simulink model "Parte2_Controlador"  (R2024a)
settings: Solver=VariableStepAuto  StartTime=0.0  StopTime=20  RelTol=1e-3
settings Model: Creator=salio  LastModifiedBy=Marco
settings SolverCC: MaxConsecutiveMinStep=10  ZeroCrossAlgorithm=Adaptive
settings OptimizationCC: ReuseModelBlockBuffer=off
settings DebuggingCC: SignalInfNanChecking=error  IgnoredZcDiagnostic=none
settings RTWCC: GPUComputeCapability=3.5

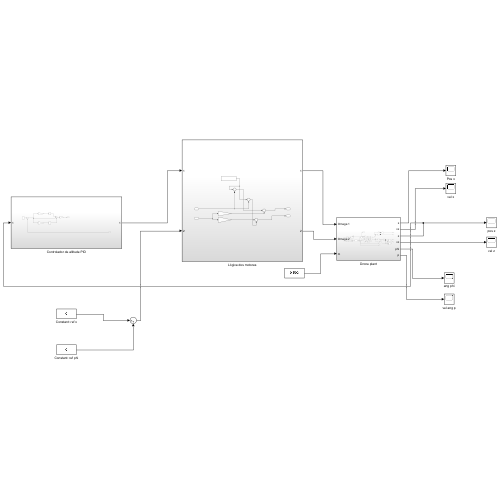
[thumbnail: Simulink's stored preview of the top-level diagram]
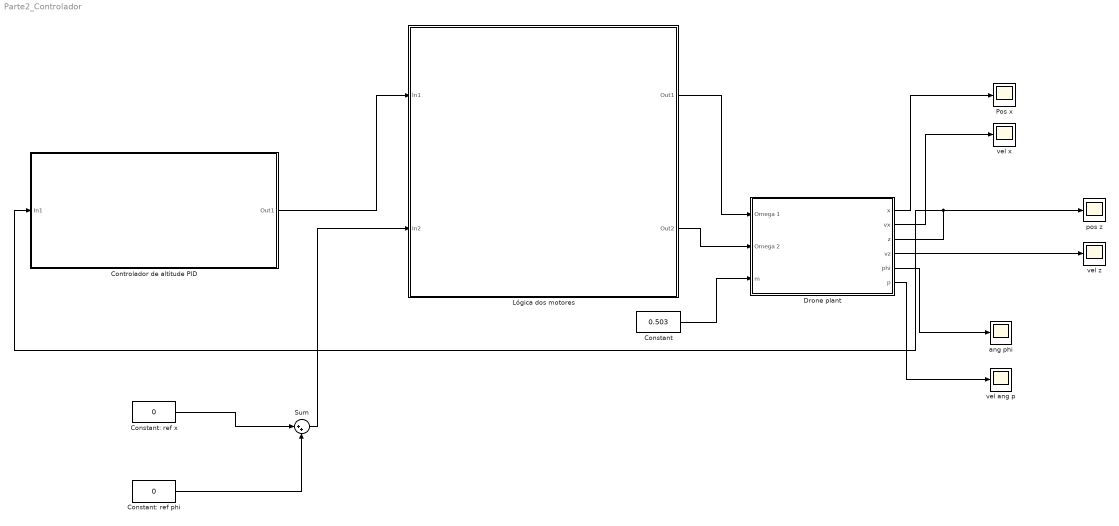
== system Parte2_Controlador ==
  Constant : Constant  Value=0.503
  Constant: ref phi : Constant  Value=0
  Constant: ref x : Constant  Value=0
  Controlador de altitude PID : Subsystem
  Drone plant : Subsystem
  Lógica dos motores : Subsystem
  Pos x : Scope
  Sum : Sum  Inputs=|++
  ang phi : Scope
  pos z : Scope
  vel ang p : Scope
  vel x : Scope
  vel z : Scope
  wires:
  Constant/1 -> Drone plant/3(m)
  Drone plant/1(x) -> Pos x/1
  Drone plant/2(vx) -> vel x/1
  Drone plant/5(phi) -> ang phi/1
  Drone plant/6(p) -> vel ang p/1
  Drone plant/3(z) -> Controlador de altitude PID/1(In1), pos z/1
  Drone plant/4(vz) -> vel z/1
  Sum/1 -> Lógica dos motores/2(In2)
  Lógica dos motores/1(Out1) -> Drone plant/1(Omega 1)
  Lógica dos motores/2(Out2) -> Drone plant/2(Omega 2)
  Controlador de altitude PID/1(Out1) -> Lógica dos motores/1(In1)
  Constant: ref x/1 -> Sum/1
  Constant: ref phi/1 -> Sum/2

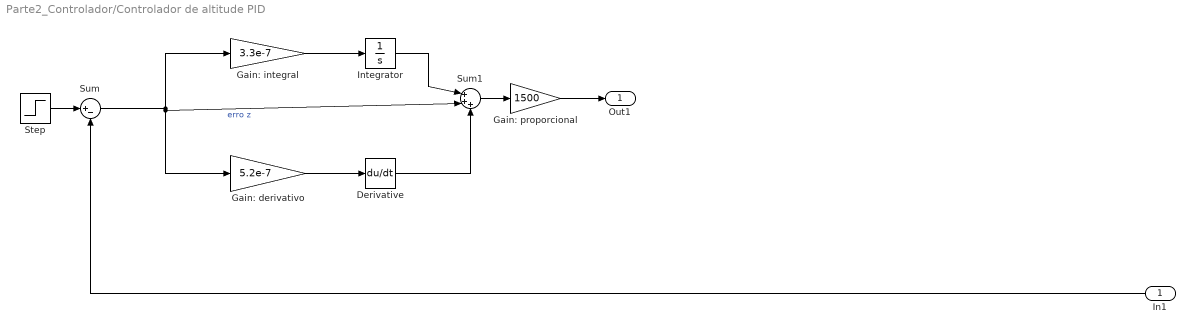
== system Parte2_Controlador/Controlador de altitude PID ==
  In1 : Inport
  Derivative : Derivative
  Gain: derivativo : Gain  Gain=5.2e-7
  Gain: integral : Gain  Gain=3.3e-7
  Gain: proporcional : Gain  Gain=1500
  Integrator : Integrator
  Step : Step  After=5  SampleTime=0
  Sum : Sum  Inputs=|+-
  Sum1 : Sum  Inputs=|+++
  Out1 : Outport
  wires:
  In1/1 -> Sum/2
  Step/1 -> Sum/1
  Gain: integral/1 -> Integrator/1
  Sum/1 -> Gain: derivativo/1, Sum1/2, Gain: integral/1  "erro z"
  Gain: derivativo/1 -> Derivative/1
  Integrator/1 -> Sum1/1
  Derivative/1 -> Sum1/3
  Sum1/1 -> Gain: proporcional/1
  Gain: proporcional/1 -> Out1/1

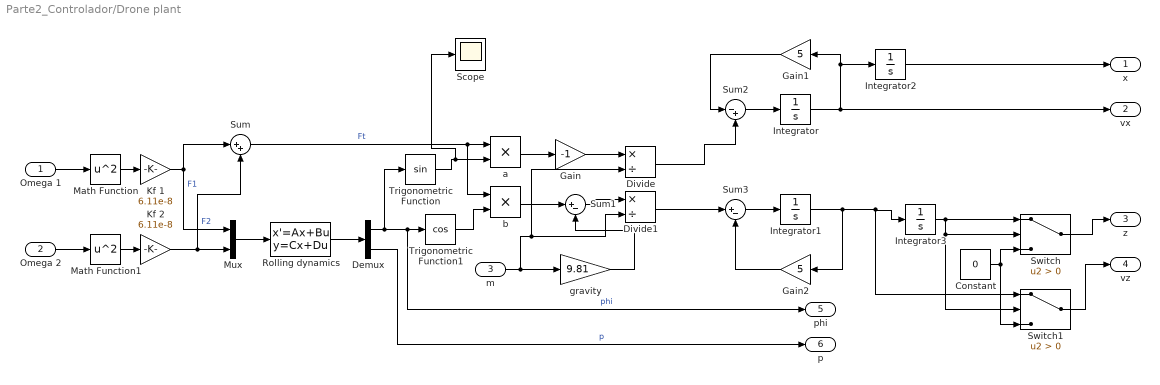
== system Parte2_Controlador/Drone plant ==
  Omega 1 : Inport
  Omega 2 : Inport  Port=2
  m : Inport  Port=3
  Constant : Constant  Value=0
  Demux : Demux  Outputs=2
  Divide : Product  Inputs=*/
  Divide1 : Product  Inputs=*/
  Gain : Gain  Gain=-1
  Gain1 : Gain  Gain=5
  Gain2 : Gain  Gain=5
  Integrator{,1..3} (4 alike) : Integrator
  Kf 1 : Gain  Gain=6.11e-8
  Kf 2 : Gain  Gain=6.11e-8
  Math Function : Math  Operator=square
  Math Function1 : Math  Operator=square
  Mux : Mux  Inputs=2
  Rolling dynamics : StateSpace  A=[0 1; 0 -1800]  B=[0 0; 110.8 -110.8]  C=[1 0; 0 1]  D=[0 0; 0 0]  InitialCondition=0
  Scope : Scope
  Sum : Sum  Inputs=|++
  Sum1 : Sum  Inputs=|+-
  Sum2 : Sum  Inputs=|-+
  Sum3 : Sum  Inputs=|+-
  Switch : Switch  Criteria=u2 > Threshold  SaturateOnIntegerOverflow=off  InputSameDT=off
  Switch1 : Switch  Criteria=u2 > Threshold  SaturateOnIntegerOverflow=off  InputSameDT=off
  Trigonometric Function : Trigonometry
  Trigonometric Function1 : Trigonometry  Operator=cos
  a : Product
  b : Product
  gravity : Gain  Gain=9.81
  x : Outport
  vx : Outport  Port=2
  z : Outport  Port=3
  vz : Outport  Port=4
  phi : Outport  Port=5
  p : Outport  Port=6
  wires:
  Demux/1 -> phi/1, Trigonometric Function1/1, Trigonometric Function/1  "phi"
  Omega 2/1 -> Math Function1/1
  Kf 2/1 -> Mux/2, Sum/2  "F2"
  Kf 1/1 -> Mux/1, Sum/1  "F1"
  Demux/2 -> p/1  "p"
  Trigonometric Function/1 -> Scope/1, a/2
  Math Function/1 -> Kf 1/1
  Omega 1/1 -> Math Function/1
  Mux/1 -> Rolling dynamics/1
  Rolling dynamics/1 -> Demux/1
  Sum/1 -> b/1, a/1  "Ft"
  Trigonometric Function1/1 -> b/2
  Math Function1/1 -> Kf 2/1
  Switch/1 -> z/1
  a/1 -> Gain/1
  Gain/1 -> Divide/1
  Divide/1 -> Sum2/2
  Integrator2/1 -> x/1
  Divide1/1 -> Sum3/1
  Integrator3/1 -> Switch1/2, Switch/2, Switch/1
  m/1 -> Divide1/2, Divide/2, gravity/1
  b/1 -> Sum1/1
  gravity/1 -> Sum1/2
  Sum1/1 -> Divide1/1
  Integrator/1 -> vx/1, Gain1/1, Integrator2/1
  Gain1/1 -> Sum2/1
  Sum2/1 -> Integrator/1
  Sum3/1 -> Integrator1/1
  Constant/1 -> Switch1/3, Switch/3
  Switch1/1 -> vz/1
  Integrator1/1 -> Gain2/1, Switch1/1, Integrator3/1
  Gain2/1 -> Sum3/2

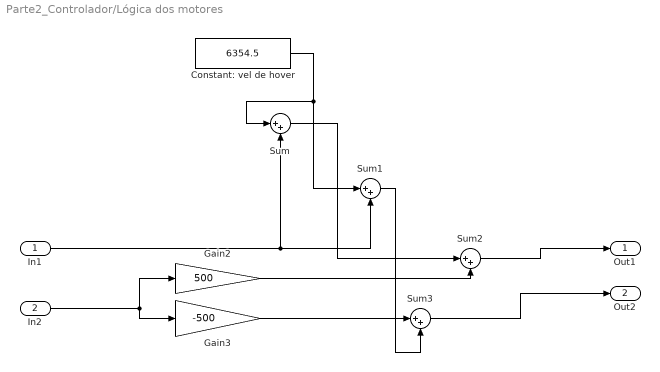
== system Parte2_Controlador/Lógica dos motores ==
  In1 : Inport
  In2 : Inport  Port=2
  Constant: vel de hover : Constant  Value=6354.5
  Gain2 : Gain  Gain=500
  Gain3 : Gain  Gain=-500
  Sum{,1..3} (4 alike) : Sum  Inputs=|++
  Out1 : Outport
  Out2 : Outport  Port=2
  wires:
  In2/1 -> Gain3/1, Gain2/1
  Constant: vel de hover/1 -> Sum1/1, Sum/1
  Sum1/1 -> Sum3/2
  Sum/1 -> Sum2/1
  Gain2/1 -> Sum2/2
  Gain3/1 -> Sum3/1
  Sum2/1 -> Out1/1
  Sum3/1 -> Out2/1
  In1/1 -> Sum1/2, Sum/2
